simulink model "stm32f4_rtc_configure_demo"  (Simulink 7.3)
settings: Solver=FixedStepDiscrete  SolverMode=SingleTasking  StartTime=0.0  StopTime=10.0  RelTol=1e-3
PreLoadFcn:
  | waijung.modelPreload; % Required for working with Waijung Blockset. Do not remove.
undefined symbols (not defined in the file): HSEOSC, Link, LQFP176, ST, STM32F417IG
libraries: simulink x54, amg_high_precision_rtc x5, stm32f4_io_lib x2, stm32f4_device_config_lib x1
(part 3 of 3)

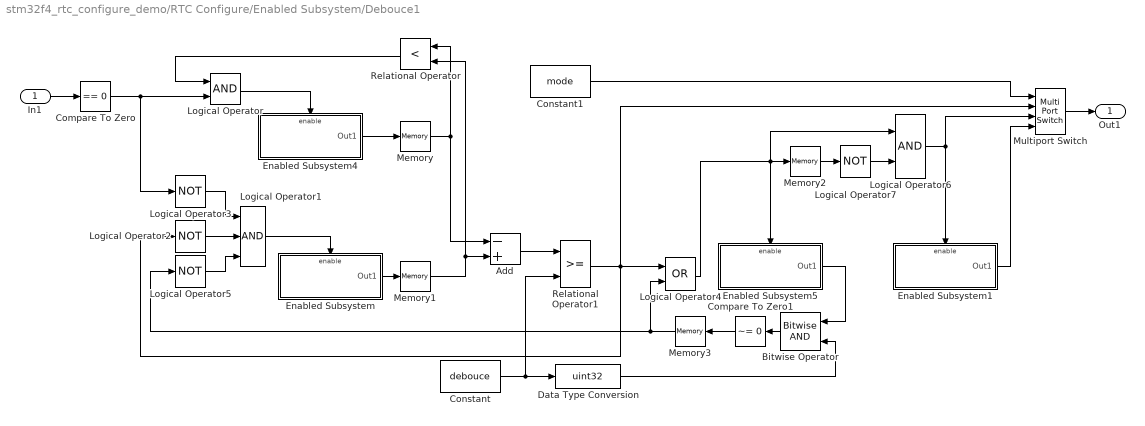
== system stm32f4_rtc_configure_demo/RTC Configure/Enabled Subsystem/Debouce1 ==
  In1 : Inport  OutDataType=fixdt(1, 16)  OutScaling=2^0
  Add : Sum  Inputs=-+  OutDataTypeMode=int32  OutDataType=fixdt(1, 16)  OutScaling=2^-10  OutDataTypeStr=int32
  Bitwise Operator : simulink/Logic and Bit Operations/Bitwise Operator  logicop=AND  UseBitMask=off  NumInputPorts=2  BitMask=debouce  BitMaskRealWorld=Stored Integer
  Compare To Zero : simulink/Logic and Bit Operations/Compare To Zero  SystemSampleTime=-1  relop===  LogicOutDataTypeMode=uint8  ZeroCross=off
  Compare To Zero1 : simulink/Logic and Bit Operations/Compare To Zero  SystemSampleTime=-1  relop=~=  LogicOutDataTypeMode=boolean  ZeroCross=off
  Constant : Constant  Value=debouce  OutDataTypeMode=int32  OutDataType=fixdt(1, 16)  OutScaling=2^0  OutDataTypeStr=int32
  Constant1 : Constant  Value=mode  OutDataTypeMode=int32  OutDataType=fixdt(1, 16)  OutScaling=2^0  OutDataTypeStr=int32
  Data Type Conversion : DataTypeConversion  OutDataTypeMode=uint32  OutDataType=fixdt(1, 16)  OutScaling=2^0  OutDataTypeStr=uint32
  Enabled Subsystem : Subsystem  TreatAsAtomicUnit=on
  Enabled Subsystem1 : Subsystem  TreatAsAtomicUnit=on
  Enabled Subsystem4 : Subsystem  TreatAsAtomicUnit=on
  Enabled Subsystem5 : Subsystem  TreatAsAtomicUnit=on
  Logical Operator : Logic  AllPortsSameDT=off  OutDataTypeMode=boolean  LogicDataType=fixdt(0, 8)  OutDataTypeStr=boolean
  Logical Operator1 : Logic  Inputs=3  AllPortsSameDT=off  OutDataTypeMode=boolean  LogicDataType=fixdt(0, 8)  OutDataTypeStr=boolean
  Logical Operator{2..3,5,7} (4 alike) : Logic  Operator=NOT  AllPortsSameDT=off  OutDataTypeMode=boolean  LogicDataType=fixdt(0, 8)  OutDataTypeStr=boolean
  Logical Operator4 : Logic  Operator=OR  AllPortsSameDT=off  OutDataTypeMode=boolean  LogicDataType=fixdt(0, 8)  OutDataTypeStr=boolean
  Logical Operator6 : Logic  AllPortsSameDT=off  OutDataTypeMode=boolean  LogicDataType=fixdt(0, 8)  OutDataTypeStr=boolean
  Memory{,1..3} (4 alike) : Memory  LinearizeMemory=on
  Multiport Switch : MultiPortSwitch  OutDataType=fixdt(1, 16)  OutScaling=2^0
  Relational Operator : RelationalOperator  Operator=<  LogicOutDataTypeMode=boolean  LogicDataType=fixdt(0, 8)  OutDataTypeStr=boolean
  Relational Operator1 : RelationalOperator  LogicOutDataTypeMode=boolean  LogicDataType=fixdt(0, 8)  OutDataTypeStr=boolean  InputSameDT=on
  Out1 : Outport  OutDataType=fixdt(1, 16)  OutScaling=2^0
  wires:
  Constant1/1 -> Multiport Switch/1
  Multiport Switch/1 -> Out1/1
  Data Type Conversion/1 -> Bitwise Operator/2
  Enabled Subsystem1/1(Out1) -> Multiport Switch/4
  Logical Operator6/1 -> Enabled Subsystem1/Enable, Multiport Switch/3
  In1/1 -> Compare To Zero/1
  Enabled Subsystem/1(Out1) -> Memory1/1
  Enabled Subsystem4/1(Out1) -> Memory/1
  Memory/1 -> Relational Operator/1, Add/1
  Memory1/1 -> Add/2, Relational Operator/2
  Compare To Zero/1 -> Logical Operator/2, Logical Operator3/1
  Logical Operator/1 -> Enabled Subsystem4/Enable
  Relational Operator/1 -> Logical Operator/1
  Add/1 -> Relational Operator1/1
  Constant/1 -> Data Type Conversion/1, Relational Operator1/2
  Logical Operator2/1 -> Logical Operator1/2
  Memory3/1 -> Logical Operator4/2, Logical Operator5/1
  Logical Operator5/1 -> Logical Operator1/3
  Logical Operator3/1 -> Logical Operator1/1
  Compare To Zero1/1 -> Memory3/1
  Bitwise Operator/1 -> Compare To Zero1/1
  Enabled Subsystem5/1(Out1) -> Bitwise Operator/1
  Logical Operator4/1 -> Enabled Subsystem5/Enable, Memory2/1, Logical Operator6/1
  Memory2/1 -> Logical Operator7/1
  Logical Operator7/1 -> Logical Operator6/2
  Relational Operator1/1 -> Multiport Switch/2, Logical Operator4/1, Logical Operator2/1
  Logical Operator1/1 -> Enabled Subsystem/Enable

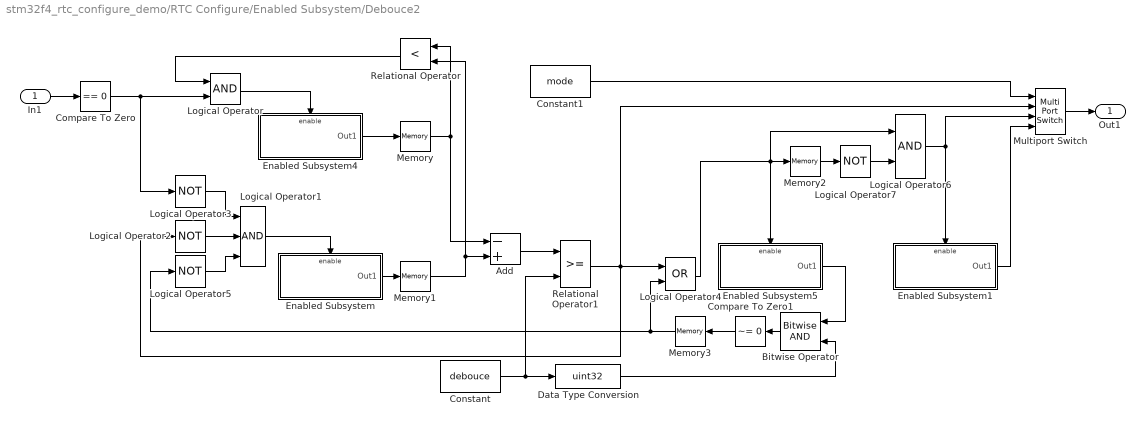
== system stm32f4_rtc_configure_demo/RTC Configure/Enabled Subsystem/Debouce2 ==
  In1 : Inport  OutDataType=fixdt(1, 16)  OutScaling=2^0
  Add : Sum  Inputs=-+  OutDataTypeMode=int32  OutDataType=fixdt(1, 16)  OutScaling=2^-10  OutDataTypeStr=int32
  Bitwise Operator : simulink/Logic and Bit Operations/Bitwise Operator  logicop=AND  UseBitMask=off  NumInputPorts=2  BitMask=debouce  BitMaskRealWorld=Stored Integer
  Compare To Zero : simulink/Logic and Bit Operations/Compare To Zero  SystemSampleTime=-1  relop===  LogicOutDataTypeMode=uint8  ZeroCross=off
  Compare To Zero1 : simulink/Logic and Bit Operations/Compare To Zero  SystemSampleTime=-1  relop=~=  LogicOutDataTypeMode=boolean  ZeroCross=off
  Constant : Constant  Value=debouce  OutDataTypeMode=int32  OutDataType=fixdt(1, 16)  OutScaling=2^0  OutDataTypeStr=int32
  Constant1 : Constant  Value=mode  OutDataTypeMode=int32  OutDataType=fixdt(1, 16)  OutScaling=2^0  OutDataTypeStr=int32
  Data Type Conversion : DataTypeConversion  OutDataTypeMode=uint32  OutDataType=fixdt(1, 16)  OutScaling=2^0  OutDataTypeStr=uint32
  Enabled Subsystem : Subsystem  TreatAsAtomicUnit=on
  Enabled Subsystem1 : Subsystem  TreatAsAtomicUnit=on
  Enabled Subsystem4 : Subsystem  TreatAsAtomicUnit=on
  Enabled Subsystem5 : Subsystem  TreatAsAtomicUnit=on
  Logical Operator : Logic  AllPortsSameDT=off  OutDataTypeMode=boolean  LogicDataType=fixdt(0, 8)  OutDataTypeStr=boolean
  Logical Operator1 : Logic  Inputs=3  AllPortsSameDT=off  OutDataTypeMode=boolean  LogicDataType=fixdt(0, 8)  OutDataTypeStr=boolean
  Logical Operator{2..3,5,7} (4 alike) : Logic  Operator=NOT  AllPortsSameDT=off  OutDataTypeMode=boolean  LogicDataType=fixdt(0, 8)  OutDataTypeStr=boolean
  Logical Operator4 : Logic  Operator=OR  AllPortsSameDT=off  OutDataTypeMode=boolean  LogicDataType=fixdt(0, 8)  OutDataTypeStr=boolean
  Logical Operator6 : Logic  AllPortsSameDT=off  OutDataTypeMode=boolean  LogicDataType=fixdt(0, 8)  OutDataTypeStr=boolean
  Memory{,1..3} (4 alike) : Memory  LinearizeMemory=on
  Multiport Switch : MultiPortSwitch  OutDataType=fixdt(1, 16)  OutScaling=2^0
  Relational Operator : RelationalOperator  Operator=<  LogicOutDataTypeMode=boolean  LogicDataType=fixdt(0, 8)  OutDataTypeStr=boolean
  Relational Operator1 : RelationalOperator  LogicOutDataTypeMode=boolean  LogicDataType=fixdt(0, 8)  OutDataTypeStr=boolean  InputSameDT=on
  Out1 : Outport  OutDataType=fixdt(1, 16)  OutScaling=2^0
  wires:
  Constant1/1 -> Multiport Switch/1
  Multiport Switch/1 -> Out1/1
  Data Type Conversion/1 -> Bitwise Operator/2
  Enabled Subsystem1/1(Out1) -> Multiport Switch/4
  Logical Operator6/1 -> Enabled Subsystem1/Enable, Multiport Switch/3
  In1/1 -> Compare To Zero/1
  Enabled Subsystem/1(Out1) -> Memory1/1
  Enabled Subsystem4/1(Out1) -> Memory/1
  Memory/1 -> Relational Operator/1, Add/1
  Memory1/1 -> Add/2, Relational Operator/2
  Compare To Zero/1 -> Logical Operator/2, Logical Operator3/1
  Logical Operator/1 -> Enabled Subsystem4/Enable
  Relational Operator/1 -> Logical Operator/1
  Add/1 -> Relational Operator1/1
  Constant/1 -> Data Type Conversion/1, Relational Operator1/2
  Logical Operator2/1 -> Logical Operator1/2
  Memory3/1 -> Logical Operator4/2, Logical Operator5/1
  Logical Operator5/1 -> Logical Operator1/3
  Logical Operator3/1 -> Logical Operator1/1
  Compare To Zero1/1 -> Memory3/1
  Bitwise Operator/1 -> Compare To Zero1/1
  Enabled Subsystem5/1(Out1) -> Bitwise Operator/1
  Logical Operator4/1 -> Enabled Subsystem5/Enable, Memory2/1, Logical Operator6/1
  Memory2/1 -> Logical Operator7/1
  Logical Operator7/1 -> Logical Operator6/2
  Relational Operator1/1 -> Multiport Switch/2, Logical Operator4/1, Logical Operator2/1
  Logical Operator1/1 -> Enabled Subsystem/Enable

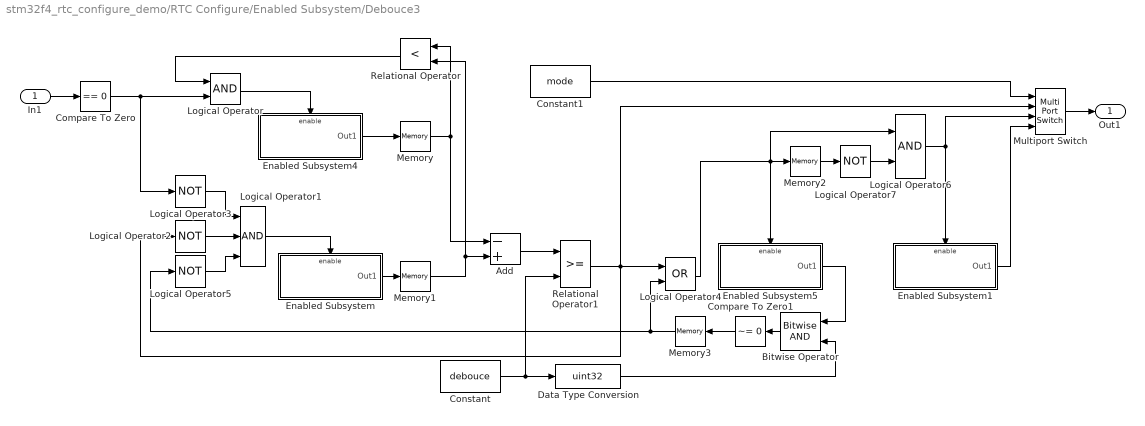
== system stm32f4_rtc_configure_demo/RTC Configure/Enabled Subsystem/Debouce3 ==
  In1 : Inport  OutDataType=fixdt(1, 16)  OutScaling=2^0
  Add : Sum  Inputs=-+  OutDataTypeMode=int32  OutDataType=fixdt(1, 16)  OutScaling=2^-10  OutDataTypeStr=int32
  Bitwise Operator : simulink/Logic and Bit Operations/Bitwise Operator  logicop=AND  UseBitMask=off  NumInputPorts=2  BitMask=debouce  BitMaskRealWorld=Stored Integer
  Compare To Zero : simulink/Logic and Bit Operations/Compare To Zero  SystemSampleTime=-1  relop===  LogicOutDataTypeMode=uint8  ZeroCross=off
  Compare To Zero1 : simulink/Logic and Bit Operations/Compare To Zero  SystemSampleTime=-1  relop=~=  LogicOutDataTypeMode=boolean  ZeroCross=off
  Constant : Constant  Value=debouce  OutDataTypeMode=int32  OutDataType=fixdt(1, 16)  OutScaling=2^0  OutDataTypeStr=int32
  Constant1 : Constant  Value=mode  OutDataTypeMode=int32  OutDataType=fixdt(1, 16)  OutScaling=2^0  OutDataTypeStr=int32
  Data Type Conversion : DataTypeConversion  OutDataTypeMode=uint32  OutDataType=fixdt(1, 16)  OutScaling=2^0  OutDataTypeStr=uint32
  Enabled Subsystem : Subsystem  TreatAsAtomicUnit=on
  Enabled Subsystem1 : Subsystem  TreatAsAtomicUnit=on
  Enabled Subsystem4 : Subsystem  TreatAsAtomicUnit=on
  Enabled Subsystem5 : Subsystem  TreatAsAtomicUnit=on
  Logical Operator : Logic  AllPortsSameDT=off  OutDataTypeMode=boolean  LogicDataType=fixdt(0, 8)  OutDataTypeStr=boolean
  Logical Operator1 : Logic  Inputs=3  AllPortsSameDT=off  OutDataTypeMode=boolean  LogicDataType=fixdt(0, 8)  OutDataTypeStr=boolean
  Logical Operator{2..3,5,7} (4 alike) : Logic  Operator=NOT  AllPortsSameDT=off  OutDataTypeMode=boolean  LogicDataType=fixdt(0, 8)  OutDataTypeStr=boolean
  Logical Operator4 : Logic  Operator=OR  AllPortsSameDT=off  OutDataTypeMode=boolean  LogicDataType=fixdt(0, 8)  OutDataTypeStr=boolean
  Logical Operator6 : Logic  AllPortsSameDT=off  OutDataTypeMode=boolean  LogicDataType=fixdt(0, 8)  OutDataTypeStr=boolean
  Memory{,1..3} (4 alike) : Memory  LinearizeMemory=on
  Multiport Switch : MultiPortSwitch  OutDataType=fixdt(1, 16)  OutScaling=2^0
  Relational Operator : RelationalOperator  Operator=<  LogicOutDataTypeMode=boolean  LogicDataType=fixdt(0, 8)  OutDataTypeStr=boolean
  Relational Operator1 : RelationalOperator  LogicOutDataTypeMode=boolean  LogicDataType=fixdt(0, 8)  OutDataTypeStr=boolean  InputSameDT=on
  Out1 : Outport  OutDataType=fixdt(1, 16)  OutScaling=2^0
  wires:
  Constant1/1 -> Multiport Switch/1
  Multiport Switch/1 -> Out1/1
  Data Type Conversion/1 -> Bitwise Operator/2
  Enabled Subsystem1/1(Out1) -> Multiport Switch/4
  Logical Operator6/1 -> Enabled Subsystem1/Enable, Multiport Switch/3
  In1/1 -> Compare To Zero/1
  Enabled Subsystem/1(Out1) -> Memory1/1
  Enabled Subsystem4/1(Out1) -> Memory/1
  Memory/1 -> Relational Operator/1, Add/1
  Memory1/1 -> Add/2, Relational Operator/2
  Compare To Zero/1 -> Logical Operator/2, Logical Operator3/1
  Logical Operator/1 -> Enabled Subsystem4/Enable
  Relational Operator/1 -> Logical Operator/1
  Add/1 -> Relational Operator1/1
  Constant/1 -> Data Type Conversion/1, Relational Operator1/2
  Logical Operator2/1 -> Logical Operator1/2
  Memory3/1 -> Logical Operator4/2, Logical Operator5/1
  Logical Operator5/1 -> Logical Operator1/3
  Logical Operator3/1 -> Logical Operator1/1
  Compare To Zero1/1 -> Memory3/1
  Bitwise Operator/1 -> Compare To Zero1/1
  Enabled Subsystem5/1(Out1) -> Bitwise Operator/1
  Logical Operator4/1 -> Enabled Subsystem5/Enable, Memory2/1, Logical Operator6/1
  Memory2/1 -> Logical Operator7/1
  Logical Operator7/1 -> Logical Operator6/2
  Relational Operator1/1 -> Multiport Switch/2, Logical Operator4/1, Logical Operator2/1
  Logical Operator1/1 -> Enabled Subsystem/Enable

== system stm32f4_rtc_configure_demo/RTC Configure/Enabled Subsystem/Generate Mode ID ==
  note: # check unused state
  In1 : Inport
  Compare To Constant : simulink/Logic and Bit Operations/Compare To Constant  SystemSampleTime=-1  relop=>  const=5  LogicOutDataTypeMode=boolean  ZeroCross=off
  Enabled Subsystem2 : Subsystem  TreatAsAtomicUnit=on
  Logical Operator : Logic  Operator=OR  AllPortsSameDT=off  OutDataTypeMode=boolean  LogicDataType=fixdt(0, 8)  OutDataTypeStr=boolean
  Unit Delay : UnitDelay  SampleTime=-1
  Out1 : Outport
  wires:
  In1/1 -> Logical Operator/2
  Unit Delay/1 -> Compare To Constant/1
  Compare To Constant/1 -> Logical Operator/1
  Logical Operator/1 -> Enabled Subsystem2/Enable
  Enabled Subsystem2/1(Out1) -> Out1/1, Unit Delay/1

== system stm32f4_rtc_configure_demo/RTC Configure/Enabled Subsystem/Subsystem ==
  Up : Inport
  Down : Inport  Port=2
  Adjust State : Inport  Port=3
  Enable : EnablePort
  Enabled Subsystem : Subsystem  TreatAsAtomicUnit=on
  RTC Date Read : S-Function  FunctionName=stm32f4_rtc  Parameters=inputtypearray,outputtypearray,confstr,sampletime,sampletimestr,blockid  EnableBusSupport=off  mask(stm32f4_rtc){configuration=DateRead, clocksource=LSE (32.768kHz), dataformat=BIN, hourformat=HourFormat_24, inputtypearray=[0], outputtypearray=[4 3 3 3 3], confstr=["DateRead","LSE (32.768kHz)","BIN","HourFormat_24"], sampletime=0.01, sampletimestr=0.01, blockid=RTCConfigureEnabledSubsystemSubsystemRTCDateRead}
      mask prompts: clocksource "Clock source"; dataformat "Format"; hourformat "Hour format"; inputtypearray "Input type array"; outputtypearray "Output type array"; confstr "Configuration string"; sampletime "Sample time (sec)"; sampletimestr "Compiled sample time (sec) in string"
      mask init:
      | stm32f4_rtc_callback('init');
      mask Help: web(fullfile(waijungdocroot,'stm32f4_rtc_setup.htm'), '-browser')
      mask StyleString: popup(Setup|DateRead|TimeRead|DateWrite|TimeWrite),popup(LSE (32.768kHz)|LSI),popup(BCD|BIN),popup(HourFormat_24|HourFormat_12),edit,edit,edit,edit,edit,edit
      mask CallbackString: stm32f4_rtc_callback('configuration');||stm32f4_rtc_callback('dataformat');||||stm32f4_rtc_callback('confstr');|stm32f4_rtc_callback('sampletime');|stm32f4_rtc_callback('sampletimestr');|stm32f4_rtc_callback('blockid');
      mask Display: text(0.05, 0.5, 'Module: RTC (DateRead)\nFormat: BIN\nTs (sec): 0.01','ver','middle','hor','left');port_label('output', 1,'Day');port_label('output', 2,'Date');port_label('output', 3,'Month');port_label('output', 4,'Year');
  RTC Time Read : S-Function  FunctionName=stm32f4_rtc  Parameters=inputtypearray,outputtypearray,confstr,sampletime,sampletimestr,blockid  EnableBusSupport=off  mask(stm32f4_rtc){configuration=TimeRead, clocksource=LSE (32.768kHz), dataformat=BIN, hourformat=HourFormat_24, inputtypearray=[0], outputtypearray=[3 3 3 3], confstr=["TimeRead","LSE (32.768kHz)","BIN","HourFormat_24"], sampletime=0.01, sampletimestr=0.01, blockid=RTCConfigureEnabledSubsystemSubsystemRTCTimeRead}
      mask prompts: clocksource "Clock source"; dataformat "Format"; hourformat "Hour format"; inputtypearray "Input type array"; outputtypearray "Output type array"; confstr "Configuration string"; sampletime "Sample time (sec)"; sampletimestr "Compiled sample time (sec) in string"
      mask init:
      | stm32f4_rtc_callback('init');
      mask Help: web(fullfile(waijungdocroot,'stm32f4_rtc_setup.htm'), '-browser')
      mask StyleString: popup(Setup|DateRead|TimeRead|DateWrite|TimeWrite),popup(LSE (32.768kHz)|LSI),popup(BCD|BIN),popup(HourFormat_24|HourFormat_12),edit,edit,edit,edit,edit,edit
      mask CallbackString: stm32f4_rtc_callback('configuration');||stm32f4_rtc_callback('dataformat');||||stm32f4_rtc_callback('confstr');|stm32f4_rtc_callback('sampletime');|stm32f4_rtc_callback('sampletimestr');|stm32f4_rtc_callback('blockid');
      mask Display: text(0.05, 0.5, 'Module: RTC (TimeRead)\nFormat: BIN\nTs (sec): 0.01','ver','middle','hor','left');port_label('output', 1,'Hour');port_label('output', 2,'Minute');port_label('output', 3,'Second');
  Terminator : Terminator
  wires:
  RTC Date Read/2 -> Enabled Subsystem/1(dd)
  RTC Time Read/3 -> Enabled Subsystem/6(ss)
  RTC Time Read/2 -> Enabled Subsystem/5(mi)
  RTC Time Read/1 -> Enabled Subsystem/4(hh)
  Down/1 -> Enabled Subsystem/9(down)
  Up/1 -> Enabled Subsystem/8(up)
  Adjust State/1 -> Enabled Subsystem/7(adjust state)
  RTC Date Read/1 -> Terminator/1
  RTC Date Read/4 -> Enabled Subsystem/3(yy)
  RTC Date Read/3 -> Enabled Subsystem/2(mm)

== system stm32f4_rtc_configure_demo/RTC Configure/Enabled Subsystem/Debouce1/Enabled Subsystem ==
  Enable : EnablePort
  Counter Free-Running : simulink/Sources/Counter Free-Running  SystemSampleTime=-1  NumBits=32  tsamp=-1
  Out1 : Outport  OutDataType=fixdt(1, 16)  OutScaling=2^0  InitialOutput=0
  wires:
  Counter Free-Running/1 -> Out1/1

== system stm32f4_rtc_configure_demo/RTC Configure/Enabled Subsystem/Debouce1/Enabled Subsystem1 ==
  Enable : EnablePort
  Bitwise Operator : simulink/Logic and Bit Operations/Bitwise Operator  logicop=AND  UseBitMask=on  BitMask=1  BitMaskRealWorld=Stored Integer
  Compare To Zero : simulink/Logic and Bit Operations/Compare To Zero  SystemSampleTime=-1  relop===  LogicOutDataTypeMode=uint8  ZeroCross=off
  Counter Free-Running : simulink/Sources/Counter Free-Running  SystemSampleTime=-1  NumBits=32  tsamp=-1
  Out1 : Outport  OutDataType=fixdt(1, 16)  OutScaling=2^0  InitialOutput=0
  wires:
  Counter Free-Running/1 -> Bitwise Operator/1
  Bitwise Operator/1 -> Compare To Zero/1
  Compare To Zero/1 -> Out1/1

== system stm32f4_rtc_configure_demo/RTC Configure/Enabled Subsystem/Debouce1/Enabled Subsystem4 ==
  Enable : EnablePort
  Counter Free-Running : simulink/Sources/Counter Free-Running  SystemSampleTime=-1  NumBits=32  tsamp=-1
  Out1 : Outport  OutDataType=fixdt(1, 16)  OutScaling=2^0  InitialOutput=0
  wires:
  Counter Free-Running/1 -> Out1/1

== system stm32f4_rtc_configure_demo/RTC Configure/Enabled Subsystem/Debouce1/Enabled Subsystem5 ==
  Enable : EnablePort
  Counter Free-Running : simulink/Sources/Counter Free-Running  SystemSampleTime=-1  NumBits=32  tsamp=-1
  Out1 : Outport  OutDataType=fixdt(1, 16)  OutScaling=2^0  InitialOutput=0
  wires:
  Counter Free-Running/1 -> Out1/1

== system stm32f4_rtc_configure_demo/RTC Configure/Enabled Subsystem/Debouce2/Enabled Subsystem ==
  Enable : EnablePort
  Counter Free-Running : simulink/Sources/Counter Free-Running  SystemSampleTime=-1  NumBits=32  tsamp=-1
  Out1 : Outport  OutDataType=fixdt(1, 16)  OutScaling=2^0  InitialOutput=0
  wires:
  Counter Free-Running/1 -> Out1/1

== system stm32f4_rtc_configure_demo/RTC Configure/Enabled Subsystem/Debouce2/Enabled Subsystem1 ==
  Enable : EnablePort
  Bitwise Operator : simulink/Logic and Bit Operations/Bitwise Operator  logicop=AND  UseBitMask=on  BitMask=1  BitMaskRealWorld=Stored Integer
  Compare To Zero : simulink/Logic and Bit Operations/Compare To Zero  SystemSampleTime=-1  relop===  LogicOutDataTypeMode=uint8  ZeroCross=off
  Counter Free-Running : simulink/Sources/Counter Free-Running  SystemSampleTime=-1  NumBits=32  tsamp=-1
  Out1 : Outport  OutDataType=fixdt(1, 16)  OutScaling=2^0  InitialOutput=0
  wires:
  Counter Free-Running/1 -> Bitwise Operator/1
  Bitwise Operator/1 -> Compare To Zero/1
  Compare To Zero/1 -> Out1/1

== system stm32f4_rtc_configure_demo/RTC Configure/Enabled Subsystem/Debouce2/Enabled Subsystem4 ==
  Enable : EnablePort
  Counter Free-Running : simulink/Sources/Counter Free-Running  SystemSampleTime=-1  NumBits=32  tsamp=-1
  Out1 : Outport  OutDataType=fixdt(1, 16)  OutScaling=2^0  InitialOutput=0
  wires:
  Counter Free-Running/1 -> Out1/1

== system stm32f4_rtc_configure_demo/RTC Configure/Enabled Subsystem/Debouce2/Enabled Subsystem5 ==
  Enable : EnablePort
  Counter Free-Running : simulink/Sources/Counter Free-Running  SystemSampleTime=-1  NumBits=32  tsamp=-1
  Out1 : Outport  OutDataType=fixdt(1, 16)  OutScaling=2^0  InitialOutput=0
  wires:
  Counter Free-Running/1 -> Out1/1

== system stm32f4_rtc_configure_demo/RTC Configure/Enabled Subsystem/Debouce3/Enabled Subsystem ==
  Enable : EnablePort
  Counter Free-Running : simulink/Sources/Counter Free-Running  SystemSampleTime=-1  NumBits=32  tsamp=-1
  Out1 : Outport  OutDataType=fixdt(1, 16)  OutScaling=2^0  InitialOutput=0
  wires:
  Counter Free-Running/1 -> Out1/1

== system stm32f4_rtc_configure_demo/RTC Configure/Enabled Subsystem/Debouce3/Enabled Subsystem1 ==
  Enable : EnablePort
  Bitwise Operator : simulink/Logic and Bit Operations/Bitwise Operator  logicop=AND  UseBitMask=on  BitMask=1  BitMaskRealWorld=Stored Integer
  Compare To Zero : simulink/Logic and Bit Operations/Compare To Zero  SystemSampleTime=-1  relop===  LogicOutDataTypeMode=uint8  ZeroCross=off
  Counter Free-Running : simulink/Sources/Counter Free-Running  SystemSampleTime=-1  NumBits=32  tsamp=-1
  Out1 : Outport  OutDataType=fixdt(1, 16)  OutScaling=2^0  InitialOutput=0
  wires:
  Counter Free-Running/1 -> Bitwise Operator/1
  Bitwise Operator/1 -> Compare To Zero/1
  Compare To Zero/1 -> Out1/1

== system stm32f4_rtc_configure_demo/RTC Configure/Enabled Subsystem/Debouce3/Enabled Subsystem4 ==
  Enable : EnablePort
  Counter Free-Running : simulink/Sources/Counter Free-Running  SystemSampleTime=-1  NumBits=32  tsamp=-1
  Out1 : Outport  OutDataType=fixdt(1, 16)  OutScaling=2^0  InitialOutput=0
  wires:
  Counter Free-Running/1 -> Out1/1

== system stm32f4_rtc_configure_demo/RTC Configure/Enabled Subsystem/Debouce3/Enabled Subsystem5 ==
  Enable : EnablePort
  Counter Free-Running : simulink/Sources/Counter Free-Running  SystemSampleTime=-1  NumBits=32  tsamp=-1
  Out1 : Outport  OutDataType=fixdt(1, 16)  OutScaling=2^0  InitialOutput=0
  wires:
  Counter Free-Running/1 -> Out1/1

== system stm32f4_rtc_configure_demo/RTC Configure/Enabled Subsystem/Generate Mode ID/Enabled Subsystem2 ==
  Enable : EnablePort
  Bitwise Operator : simulink/Logic and Bit Operations/Bitwise Operator  logicop=AND  UseBitMask=on  BitMask=7  BitMaskRealWorld=Stored Integer
  Counter Free-Running : simulink/Sources/Counter Free-Running  SystemSampleTime=-1  NumBits=16  tsamp=-1
  Out1 : Outport  OutDataType=fixdt(1, 16)  OutScaling=2^0  InitialOutput=0
  wires:
  Bitwise Operator/1 -> Out1/1
  Counter Free-Running/1 -> Bitwise Operator/1

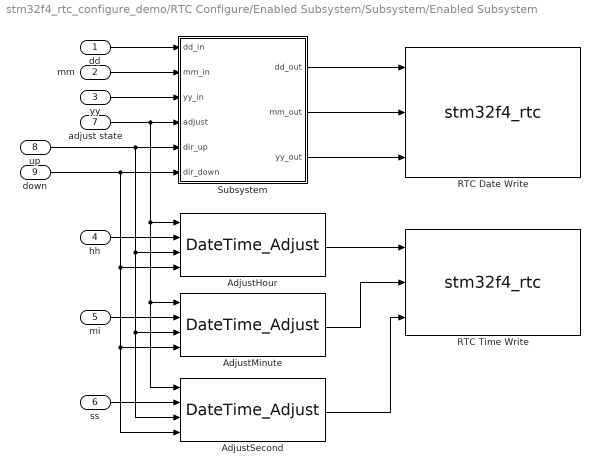
== system stm32f4_rtc_configure_demo/RTC Configure/Enabled Subsystem/Subsystem/Enabled Subsystem ==
  dd : Inport  OutDataType=fixdt(1, 16)  OutScaling=2^0
  mm : Inport  Port=2  OutDataType=fixdt(1, 16)  OutScaling=2^0
  yy : Inport  Port=3  OutDataType=fixdt(1, 16)  OutScaling=2^0
  hh : Inport  Port=4  OutDataType=fixdt(1, 16)  OutScaling=2^0
  mi : Inport  Port=5  OutDataType=fixdt(1, 16)  OutScaling=2^0
  ss : Inport  Port=6  OutDataType=fixdt(1, 16)  OutScaling=2^0
  adjust state : Inport  Port=7  OutDataType=fixdt(1, 16)  OutScaling=2^0
  up : Inport  Port=8  OutDataType=fixdt(1, 16)  OutScaling=2^0
  down : Inport  Port=9  OutDataType=fixdt(1, 16)  OutScaling=2^0
  AdjustHour : amg_high_precision_rtc/DateTime_Adjust  SystemSampleTime=-1  state=3  max=23  min=0
  AdjustMinute : amg_high_precision_rtc/DateTime_Adjust  SystemSampleTime=-1  state=4  max=59  min=0
  AdjustSecond : amg_high_precision_rtc/DateTime_Adjust  SystemSampleTime=-1  state=5  max=59  min=0
  RTC Date Write : S-Function  FunctionName=stm32f4_rtc  Parameters=inputtypearray,outputtypearray,confstr,sampletime,sampletimestr,blockid  EnableBusSupport=off  mask(stm32f4_rtc){configuration=DateWrite, clocksource=LSE (32.768kHz), dataformat=BIN, hourformat=HourFormat_24, inputtypearray=[3 -1 -1 -1], outputtypearray=[0], confstr=["DateWrite","LSE (32.768kHz)","BIN","HourFormat_24"], sampletime=0.01, sampletimestr=0.01, blockid=RTCConfigureEnabledSubsystemSubsystemEnabledSubsystemRTCDateWrite}
      mask prompts: clocksource "Clock source"; dataformat "Format"; hourformat "Hour format"; inputtypearray "Input type array"; outputtypearray "Output type array"; confstr "Configuration string"; sampletime "Sample time (sec)"; sampletimestr "Compiled sample time (sec) in string"
      mask init:
      | stm32f4_rtc_callback('init');
      mask Help: web(fullfile(waijungdocroot,'stm32f4_rtc_setup.htm'), '-browser')
      mask StyleString: popup(Setup|DateRead|TimeRead|DateWrite|TimeWrite),popup(LSE (32.768kHz)|LSI),popup(BCD|BIN),popup(HourFormat_24|HourFormat_12),edit,edit,edit,edit,edit,edit
      mask CallbackString: stm32f4_rtc_callback('configuration');||stm32f4_rtc_callback('dataformat');||||stm32f4_rtc_callback('confstr');|stm32f4_rtc_callback('sampletime');|stm32f4_rtc_callback('sampletimestr');|stm32f4_rtc_callback('blockid');
      mask Display: text(0.95, 0.5, 'Module: RTC (DateWrite)\nFormat: BIN\nTs (sec): 0.01','ver','middle','hor','right');port_label('input', 1,'Date');port_label('input', 2,'Month');port_label('input', 3,'Year');
  RTC Time Write : S-Function  FunctionName=stm32f4_rtc  Parameters=inputtypearray,outputtypearray,confstr,sampletime,sampletimestr,blockid  EnableBusSupport=off  mask(stm32f4_rtc){configuration=TimeWrite, clocksource=LSE (32.768kHz), dataformat=BIN, hourformat=HourFormat_24, inputtypearray=[3 -1 -1 -1], outputtypearray=[0], confstr=["TimeWrite","LSE (32.768kHz)","BIN","HourFormat_24"], sampletime=0.01, sampletimestr=0.01, blockid=RTCConfigureEnabledSubsystemSubsystemEnabledSubsystemRTCTimeWrite}
      mask prompts: clocksource "Clock source"; dataformat "Format"; hourformat "Hour format"; inputtypearray "Input type array"; outputtypearray "Output type array"; confstr "Configuration string"; sampletime "Sample time (sec)"; sampletimestr "Compiled sample time (sec) in string"
      mask init:
      | stm32f4_rtc_callback('init');
      mask Help: web(fullfile(waijungdocroot,'stm32f4_rtc_setup.htm'), '-browser')
      mask StyleString: popup(Setup|DateRead|TimeRead|DateWrite|TimeWrite),popup(LSE (32.768kHz)|LSI),popup(BCD|BIN),popup(HourFormat_24|HourFormat_12),edit,edit,edit,edit,edit,edit
      mask CallbackString: stm32f4_rtc_callback('configuration');||stm32f4_rtc_callback('dataformat');||||stm32f4_rtc_callback('confstr');|stm32f4_rtc_callback('sampletime');|stm32f4_rtc_callback('sampletimestr');|stm32f4_rtc_callback('blockid');
      mask Display: text(0.95, 0.5, 'Module: RTC (TimeWrite)\nFormat: BIN\nTs (sec): 0.01','ver','middle','hor','right');port_label('input', 1,'Hour');port_label('input', 2,'Minute');port_label('input', 3,'Second');
  Subsystem : Subsystem
  wires:
  AdjustMinute/1 -> RTC Time Write/2
  Subsystem/3(yy_out) -> RTC Date Write/3
  Subsystem/2(mm_out) -> RTC Date Write/2
  Subsystem/1(dd_out) -> RTC Date Write/1
  AdjustSecond/1 -> RTC Time Write/3
  AdjustHour/1 -> RTC Time Write/1
  hh/1 -> AdjustHour/2
  mi/1 -> AdjustMinute/2
  ss/1 -> AdjustSecond/2
  down/1 -> AdjustSecond/4, AdjustMinute/4, AdjustHour/4, Subsystem/6(dir_down)
  up/1 -> AdjustSecond/3, AdjustMinute/3, AdjustHour/3, Subsystem/5(dir_up)
  adjust state/1 -> AdjustSecond/1, AdjustMinute/1, AdjustHour/1, Subsystem/4(adjust)
  yy/1 -> Subsystem/3(yy_in)
  mm/1 -> Subsystem/2(mm_in)
  dd/1 -> Subsystem/1(dd_in)

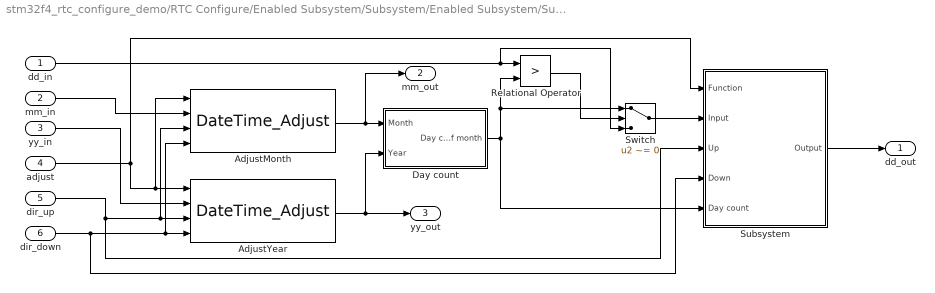
== system stm32f4_rtc_configure_demo/RTC Configure/Enabled Subsystem/Subsystem/Enabled Subsystem/Subsystem ==
  dd_in : Inport  OutDataType=fixdt(1, 16)  OutScaling=2^0
  mm_in : Inport  Port=2  OutDataType=fixdt(1, 16)  OutScaling=2^0
  yy_in : Inport  Port=3  OutDataType=fixdt(1, 16)  OutScaling=2^0
  adjust : Inport  Port=4  OutDataType=fixdt(1, 16)  OutScaling=2^0
  dir_up : Inport  Port=5  OutDataType=fixdt(1, 16)  OutScaling=2^0
  dir_down : Inport  Port=6  OutDataType=fixdt(1, 16)  OutScaling=2^0
  AdjustMonth : amg_high_precision_rtc/DateTime_Adjust  SystemSampleTime=-1  state=1  max=12  min=1
  AdjustYear : amg_high_precision_rtc/DateTime_Adjust  SystemSampleTime=-1  state=2  max=99  min=0
  Day count : Subsystem
  Relational Operator : RelationalOperator  Operator=>  LogicOutDataTypeMode=boolean  LogicDataType=fixdt(0, 8)  OutDataTypeStr=boolean
  Subsystem : Subsystem
  Switch : Switch  Criteria=u2 ~= 0  OutDataType=fixdt(1, 16)  OutScaling=2^0
  dd_out : Outport  OutDataType=fixdt(1, 16)  OutScaling=2^0
  mm_out : Outport  Port=2  OutDataType=fixdt(1, 16)  OutScaling=2^0
  yy_out : Outport  Port=3  OutDataType=fixdt(1, 16)  OutScaling=2^0
  wires:
  Subsystem/1(Output) -> dd_out/1
  Relational Operator/1 -> Switch/2
  Day count/1(Day count of month) -> Subsystem/5(Day count), Switch/1, Relational Operator/2
  Switch/1 -> Subsystem/2(Input)
  dd_in/1 -> Switch/3, Relational Operator/1
  AdjustMonth/1 -> mm_out/1, Day count/1(Month)
  AdjustYear/1 -> yy_out/1, Day count/2(Year)
  mm_in/1 -> AdjustMonth/2
  yy_in/1 -> AdjustYear/2
  adjust/1 -> Subsystem/1(Function), AdjustMonth/1, AdjustYear/1
  dir_up/1 -> Subsystem/3(Up), AdjustMonth/3, AdjustYear/3
  dir_down/1 -> Subsystem/4(Down), AdjustMonth/4, AdjustYear/4

== system stm32f4_rtc_configure_demo/RTC Configure/Enabled Subsystem/Subsystem/Enabled Subsystem/Subsystem/Day count ==
  Month : Inport  OutDataType=fixdt(1, 16)  OutScaling=2^0
  Year : Inport  Port=2  OutDataType=fixdt(1, 16)  OutScaling=2^0
  Constant : Constant  Value=30  OutDataTypeMode=uint8  OutDataType=fixdt(1, 16)  OutScaling=2^0  OutDataTypeStr=uint8
  Constant1 : Constant  Value=31  OutDataTypeMode=uint8  OutDataType=fixdt(1, 16)  OutScaling=2^0  OutDataTypeStr=uint8
  Days 30 : Subsystem
  Subsystem : Subsystem
  Switch : Switch  Criteria=u2 ~= 0  OutDataType=fixdt(1, 16)  OutScaling=2^0
  Switch1 : Switch  Criteria=u2 ~= 0  OutDataType=fixdt(1, 16)  OutScaling=2^0
  Day count of month : Outport  OutDataType=fixdt(1, 16)  OutScaling=2^0
  wires:
  Switch/1 -> Day count of month/1
  Switch1/1 -> Switch/3
  Constant1/1 -> Switch1/3
  Subsystem/2(Day count) -> Switch1/1
  Subsystem/1(Out1) -> Switch1/2
  Year/1 -> Subsystem/2(Year)
  Month/1 -> Subsystem/1(Month), Days 30/1(In1)
  Constant/1 -> Switch/1
  Days 30/1(Out1) -> Switch/2

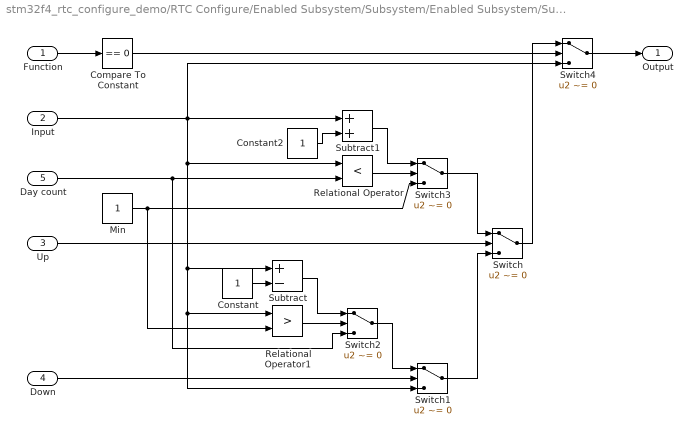
== system stm32f4_rtc_configure_demo/RTC Configure/Enabled Subsystem/Subsystem/Enabled Subsystem/Subsystem/Subsystem ==
  Function : Inport  OutDataType=fixdt(1, 16)  OutScaling=2^0
  Input : Inport  Port=2  OutDataType=fixdt(1, 16)  OutScaling=2^0
  Up : Inport  Port=3  OutDataType=fixdt(1, 16)  OutScaling=2^0
  Down : Inport  Port=4  OutDataType=fixdt(1, 16)  OutScaling=2^0
  Day count : Inport  Port=5  OutDataType=fixdt(1, 16)  OutScaling=2^0
  Compare To Constant : simulink/Logic and Bit Operations/Compare To Constant  SystemSampleTime=-1  relop===  const=0  LogicOutDataTypeMode=uint8  ZeroCross=off
  Constant : Constant  OutDataTypeMode=uint8  OutDataType=fixdt(1, 16)  OutScaling=2^0  OutDataTypeStr=uint8
  Constant2 : Constant  OutDataTypeMode=uint8  OutDataType=fixdt(1, 16)  OutScaling=2^0  OutDataTypeStr=uint8
  Min : Constant  OutDataTypeMode=uint8  OutDataType=fixdt(1, 16)  OutScaling=2^0  OutDataTypeStr=uint8
  Relational Operator : RelationalOperator  Operator=<  LogicOutDataTypeMode=boolean  LogicDataType=fixdt(0, 8)  OutDataTypeStr=boolean
  Relational Operator1 : RelationalOperator  Operator=>  LogicOutDataTypeMode=boolean  LogicDataType=fixdt(0, 8)  OutDataTypeStr=boolean
  Subtract : Sum  Inputs=+-  OutDataType=fixdt(1, 16)  OutScaling=2^-10
  Subtract1 : Sum  OutDataType=fixdt(1, 16)  OutScaling=2^-10
  Switch{,1..4} (5 alike) : Switch  Criteria=u2 ~= 0  OutDataType=fixdt(1, 16)  OutScaling=2^0
  Output : Outport  OutDataType=fixdt(1, 16)  OutScaling=2^0
  wires:
  Up/1 -> Switch/2
  Down/1 -> Switch1/2
  Switch/1 -> Switch4/1
  Compare To Constant/1 -> Switch4/2
  Switch4/1 -> Output/1
  Function/1 -> Compare To Constant/1
  Switch3/1 -> Switch/1
  Day count/1 -> Switch2/3, Relational Operator/2
  Min/1 -> Relational Operator1/2, Switch3/3
  Constant2/1 -> Subtract1/2
  Subtract1/1 -> Switch3/1
  Relational Operator/1 -> Switch3/2
  Switch2/1 -> Switch1/1
  Constant/1 -> Subtract/2
  Subtract/1 -> Switch2/1
  Relational Operator1/1 -> Switch2/2
  Input/1 -> Switch4/3, Subtract1/1, Relational Operator/1, Relational Operator1/1, Switch1/3, Subtract/1
  Switch1/1 -> Switch/3

== system stm32f4_rtc_configure_demo/RTC Configure/Enabled Subsystem/Subsystem/Enabled Subsystem/Subsystem/Day count/Days 30 ==
  In1 : Inport
  Bitwise Operator : simulink/Logic and Bit Operations/Bitwise Operator  logicop=OR  UseBitMask=off  NumInputPorts=4  BitMask=bin2dec('11011001')  BitMaskRealWorld=Stored Integer
  Compare To Constant : simulink/Logic and Bit Operations/Compare To Constant  SystemSampleTime=-1  relop===  const=6  LogicOutDataTypeMode=uint8  ZeroCross=off
  Compare To Constant1 : simulink/Logic and Bit Operations/Compare To Constant  SystemSampleTime=-1  relop===  const=4  LogicOutDataTypeMode=uint8  ZeroCross=off
  Compare To Constant2 : simulink/Logic and Bit Operations/Compare To Constant  SystemSampleTime=-1  relop===  const=9  LogicOutDataTypeMode=uint8  ZeroCross=off
  Compare To Constant3 : simulink/Logic and Bit Operations/Compare To Constant  SystemSampleTime=-1  relop===  const=11  LogicOutDataTypeMode=uint8  ZeroCross=off
  Out1 : Outport
  wires:
  Bitwise Operator/1 -> Out1/1
  In1/1 -> Compare To Constant3/1, Compare To Constant2/1, Compare To Constant/1, Compare To Constant1/1
  Compare To Constant3/1 -> Bitwise Operator/4
  Compare To Constant2/1 -> Bitwise Operator/3
  Compare To Constant/1 -> Bitwise Operator/2
  Compare To Constant1/1 -> Bitwise Operator/1

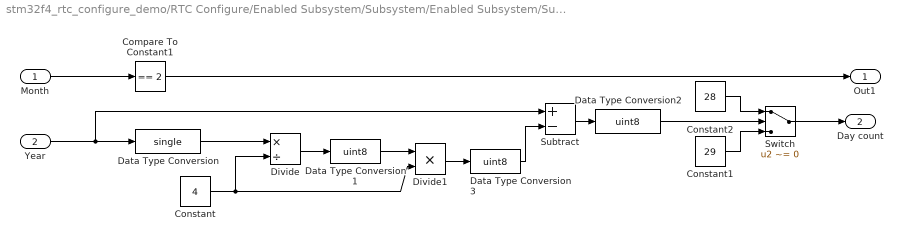
== system stm32f4_rtc_configure_demo/RTC Configure/Enabled Subsystem/Subsystem/Enabled Subsystem/Subsystem/Day count/Subsystem ==
  Month : Inport  OutDataType=fixdt(1, 16)  OutScaling=2^0
  Year : Inport  Port=2  OutDataType=fixdt(1, 16)  OutScaling=2^0
  Compare To Constant1 : simulink/Logic and Bit Operations/Compare To Constant  SystemSampleTime=-1  relop===  const=2  LogicOutDataTypeMode=uint8  ZeroCross=off
  Constant : Constant  Value=4  OutDataTypeMode=single  OutDataType=fixdt(1, 16)  OutScaling=2^0  OutDataTypeStr=single
  Constant1 : Constant  Value=29  OutDataTypeMode=uint8  OutDataType=fixdt(1, 16)  OutScaling=2^0  OutDataTypeStr=uint8
  Constant2 : Constant  Value=28  OutDataTypeMode=uint8  OutDataType=fixdt(1, 16)  OutScaling=2^0  OutDataTypeStr=uint8
  Data Type Conversion : DataTypeConversion  OutDataTypeMode=single  OutDataType=fixdt(1, 16)  OutScaling=2^0  OutDataTypeStr=single
  Data Type Conversion1 : DataTypeConversion  OutDataTypeMode=uint8  OutDataType=fixdt(1, 16)  OutScaling=2^0  OutDataTypeStr=uint8
  Data Type Conversion2 : DataTypeConversion  OutDataTypeMode=uint8  OutDataType=fixdt(1, 16)  OutScaling=2^0  OutDataTypeStr=uint8
  Data Type Conversion3 : DataTypeConversion  OutDataTypeMode=uint8  OutDataType=fixdt(1, 16)  OutScaling=2^0  OutDataTypeStr=uint8
  Divide : Product  Inputs=*/  OutDataType=fixdt(1, 16)  OutScaling=2^-10
  Divide1 : Product  Inputs=**  OutDataType=fixdt(1, 16)  OutScaling=2^-10
  Subtract : Sum  Inputs=+-  OutDataType=fixdt(1, 16)  OutScaling=2^-10
  Switch : Switch  Criteria=u2 ~= 0  OutDataType=fixdt(1, 16)  OutScaling=2^0
  Out1 : Outport  OutDataType=fixdt(1, 16)  OutScaling=2^0
  Day count : Outport  Port=2  OutDataType=fixdt(1, 16)  OutScaling=2^0
  wires:
  Data Type Conversion3/1 -> Subtract/2
  Divide1/1 -> Data Type Conversion3/1
  Data Type Conversion1/1 -> Divide1/1
  Data Type Conversion2/1 -> Switch/2
  Switch/1 -> Day count/1
  Constant2/1 -> Switch/1
  Constant1/1 -> Switch/3
  Subtract/1 -> Data Type Conversion2/1
  Divide/1 -> Data Type Conversion1/1
  Constant/1 -> Divide1/2, Divide/2
  Data Type Conversion/1 -> Divide/1
  Year/1 -> Subtract/1, Data Type Conversion/1
  Compare To Constant1/1 -> Out1/1
  Month/1 -> Compare To Constant1/1
